simulink model "Q8"  (R2016a)
settings: Solver=VariableStepAuto  StartTime=0.0  StopTime=10.0  RelTol=1e-3
values from neighbouring files (symbols this model uses):
  D2 = D'    [LabCEE.m]    (also in test.m)
  K = lqr(A, B, Qr, Rr)    [LabCEE.m]    (also in fp_ini.m; test.m)
  L = lqe(A, G, C, Qe, Re)    [LabCEE.m]    (also in fp_ini.m; test.m)
  x_0 = [0.1 0 0 0 0]'    [LabCEE.m]    (also in test.m)
undefined symbols (not defined in the file or in its folder): A, B, C, D
settings Model: Creator=ASUS  LastModifiedBy=ASUS

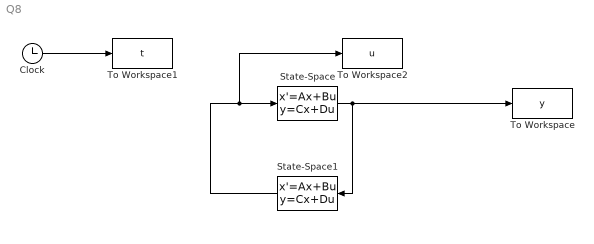
== system Q8 ==
  Clock : Clock
  State-Space : StateSpace  A=A  B=B  C=C  D=D  X0=x_0
  State-Space1 : StateSpace  A=A-B*K-L*C  B=L  C=-K  D=D2  X0=x_0
  To Workspace : ToWorkspace  VariableName=y  SampleTime=-1
  To Workspace1 : ToWorkspace  VariableName=t  SampleTime=-1
  To Workspace2 : ToWorkspace  VariableName=u  SampleTime=-1
  wires:
  Clock/1 -> To Workspace1/1
  State-Space/1 -> State-Space1/1, To Workspace/1
  State-Space1/1 -> To Workspace2/1, State-Space/1
